simulink model "orbit_propagator_matlab2023b"  (R2023b)
settings: Solver=FixedStepAuto  StartTime=0.0  StopTime=207944  FixedStep=sim_step_size  RelTol=1e-6  AbsTol=1e-7
model workspace (MAT data in the model file):
  current_year = 2025
  year = 2013
values from neighbouring files (symbols this model uses):
  alpha_acc = sqrt(0.7)    [HSat_op_setup_merged_maria.m]    (also in init_orbit_analysis_with_drag_loss.m)
  aph = 200*ones(1,7)    [init_orbit_analysis_with_drag_loss.m]
  COM = [0, 0, 0.25+0.3]    [init_orbit_analysis_with_drag_loss.m]
  ext_ENV_muEarth = 3.986005e14    (= 398600500000000)    [GEO_insertion_setup.m]    (also in HSat_op_setup.m; HSat_op_setup_merged_maria.m; init_orbit_analysis_with_drag_loss.m)
  F107 = 300    [init_orbit_analysis_with_drag_loss.m]
  P_solar = 4.56e-6    (= 4.56e-06)    [HSat_op_setup_merged_maria.m]    (also in init_orbit_analysis_with_drag_loss.m)
  perigee_vector_eci = [0, 1, 0]    [init_orbit_analysis_with_drag_loss.m]
  sim_SC_init_MoI_EOR_wet = [ ... (first row only)    [HSat_op_setup.m]    (also in HSat_op_setup_merged_maria.m; init_orbit_analysis_with_drag_loss.m)
  sim_step_size = 10    [init_orbit_analysis_with_drag_loss.m]
  sun_pointing = 1    [init_orbit_analysis_with_drag_loss.m]
  sun_pointing_SA = 0    [HSat_op_setup_merged_maria.m]    (also in init_orbit_analysis_with_drag_loss.m)
  theta = deg2rad(0)    [init_orbit_analysis_with_drag_loss.m]
undefined symbols (not defined in the file or in its folder): attitude, sun_vector_oc
libraries: aerolibutil x37, matrix_library x37, Toolbox x10, sharedtransform x10, aerolibatmos2 x1, simulink x1, simulink_extras x1
(part 2 of 3)

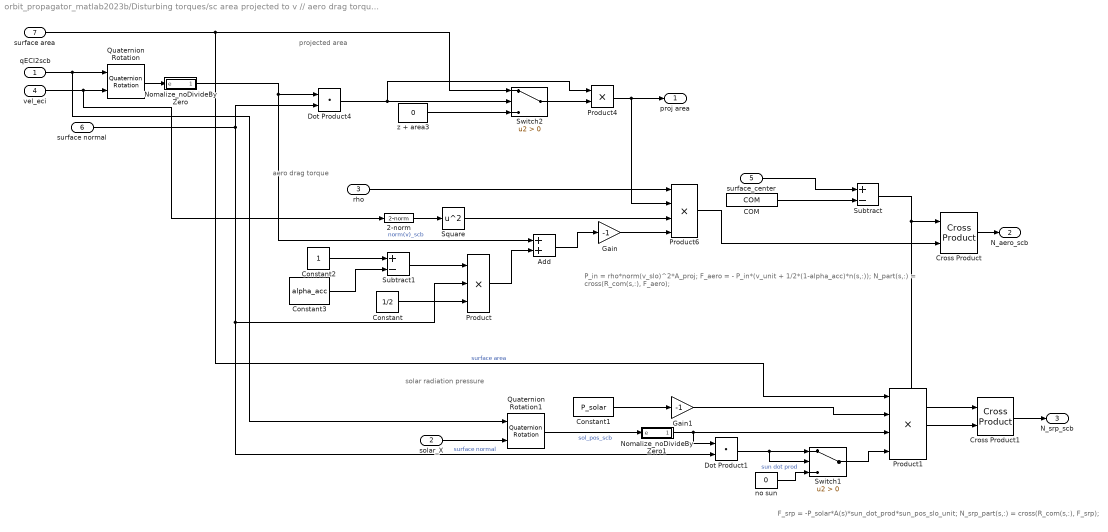
== system orbit_propagator_matlab2023b/Disturbing torques/sc area projected to v // aero drag torque // srp torque/z -6 ==
  note: projected area
  note: aero drag torque
  note: solar radiation pressure
  note: P_in = rho*norm(v_slo)^2*A_proj;
      | F_aero = - P_in*(v_unit + 1/2*(1-alpha_acc)*n(s,:));
      | N_part(s,:) = cross(R_com(s,:), F_aero);
  note: F_srp = -P_solar*A(s)*sun_dot_prod*sun_pos_slo_unit;
      | N_srp_part(s,:) = cross(R_com(s,:), F_srp);
  qECI2scb : Inport
  solar_X : Inport  Port=2
  rho : Inport  Port=3
  vel_eci : Inport  Port=4
  surface_center : Inport  Port=5
  surface normal : Inport  Port=6
  surface area : Inport  Port=7
  2-norm : Toolbox/vector blocks/2-norm  SystemSampleTime=-1  VariantActivationTime=update diagram  AllowFlexibleInterface=on  Latency=0  AutoFrameSizeCalculation=off
      settings: SourceProductName=SSC flight toolbox
  Add : Sum
  COM : Constant  Value=COM
  Constant : Constant  Value=1/2
  Constant1 : Constant  Value=P_solar
  Constant2 : Constant
  Constant3 : Constant  Value=alpha_acc
  Cross Product : matrix_library/Cross Product
  Cross Product1 : matrix_library/Cross Product
  Dot Product1 : DotProduct  OutDataTypeStr=Inherit: Inherit via internal rule
  Dot Product4 : DotProduct  OutDataTypeStr=Inherit: Inherit via internal rule
  Gain : Gain  Gain=-1
  Gain1 : Gain  Gain=-1
  Nomalize_noDivideByZero : Subsystem
      mask Display: disp('u/||u||')
  Nomalize_noDivideByZero1 : Subsystem
      mask Display: disp('u/||u||')
  Product : Product  Inputs=3
  Product1 : Product  Inputs=4
  Product4 : Product
  Product6 : Product  Inputs=4
  Quaternion Rotation : aerolibutil/Quaternion Rotation
  Quaternion Rotation1 : aerolibutil/Quaternion Rotation
  Square : Math  Operator=square
  Subtract : Sum  Inputs=+-
  Subtract1 : Sum  Inputs=+-
  Switch1 : Switch  Criteria=u2 > Threshold  SaturateOnIntegerOverflow=off  InputSameDT=off
  Switch2 : Switch  Criteria=u2 > Threshold  SaturateOnIntegerOverflow=off  InputSameDT=off
  no sun : Constant  Value=0
  z + area3 : Constant  Value=0
  proj area : Outport
  N_aero_scb : Outport  Port=2
  N_srp_scb : Outport  Port=3
  wires:
  Nomalize_noDivideByZero/1(ehat) -> Add/1, Dot Product4/1  "norm(v)_scb"
  surface area/1 -> Product1/1, Switch2/1  "surface area"
  z + area3/1 -> Switch2/3
  Switch2/1 -> Product4/2
  Product4/1 -> Product6/2, proj area/1
  Dot Product4/1 -> Product4/1, Switch2/2
  rho/1 -> Product6/1
  2-norm/1 -> Square/1
  surface normal/1 -> Dot Product4/2, Product/2, Dot Product1/2  "surface normal"
  Constant/1 -> Product/3
  Product/1 -> Add/2
  Gain/1 -> Product6/4
  Product6/1 -> Cross Product/2
  Cross Product/1 -> N_aero_scb/1
  surface_center/1 -> Subtract/1
  COM/1 -> Subtract/2
  Subtract/1 -> Cross Product1/1, Cross Product/1
  Nomalize_noDivideByZero1/1(ehat) -> Product1/3, Dot Product1/1
  Dot Product1/1 -> Switch1/2, Switch1/1  "sun dot prod"
  Constant1/1 -> Gain1/1
  Gain1/1 -> Product1/2
  Product1/1 -> Cross Product1/2
  Cross Product1/1 -> N_srp_scb/1
  vel_eci/1 -> 2-norm/1, Quaternion Rotation/2
  qECI2scb/1 -> Quaternion Rotation1/1, Quaternion Rotation/1
  Quaternion Rotation/1 -> Nomalize_noDivideByZero/1(e)
  solar_X/1 -> Quaternion Rotation1/2
  Quaternion Rotation1/1 -> Nomalize_noDivideByZero1/1(e)  "sol_pos_scb"
  Add/1 -> Gain/1
  Square/1 -> Product6/3
  Switch1/1 -> Product1/4
  no sun/1 -> Switch1/3
  Constant2/1 -> Subtract1/1
  Constant3/1 -> Subtract1/2
  Subtract1/1 -> Product/1

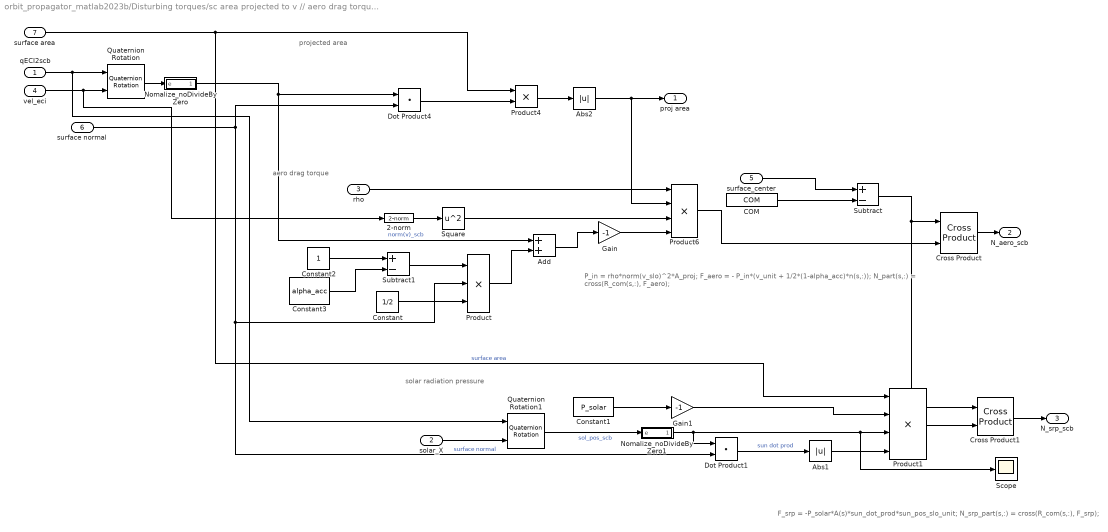
== system orbit_propagator_matlab2023b/Disturbing torques/sc area projected to v // aero drag torque // srp torque/z -7 ==
  note: projected area
  note: aero drag torque
  note: solar radiation pressure
  note: P_in = rho*norm(v_slo)^2*A_proj;
      | F_aero = - P_in*(v_unit + 1/2*(1-alpha_acc)*n(s,:));
      | N_part(s,:) = cross(R_com(s,:), F_aero);
  note: F_srp = -P_solar*A(s)*sun_dot_prod*sun_pos_slo_unit;
      | N_srp_part(s,:) = cross(R_com(s,:), F_srp);
  qECI2scb : Inport
  solar_X : Inport  Port=2
  rho : Inport  Port=3
  vel_eci : Inport  Port=4
  surface_center : Inport  Port=5
  surface normal : Inport  Port=6
  surface area : Inport  Port=7
  2-norm : Toolbox/vector blocks/2-norm  SystemSampleTime=-1  VariantActivationTime=update diagram  AllowFlexibleInterface=on  Latency=0  AutoFrameSizeCalculation=off
      settings: SourceProductName=SSC flight toolbox
  Abs1 : Abs  SaturateOnIntegerOverflow=off
  Abs2 : Abs  SaturateOnIntegerOverflow=off
  Add : Sum
  COM : Constant  Value=COM
  Constant : Constant  Value=1/2
  Constant1 : Constant  Value=P_solar
  Constant2 : Constant
  Constant3 : Constant  Value=alpha_acc
  Cross Product : matrix_library/Cross Product
  Cross Product1 : matrix_library/Cross Product
  Dot Product1 : DotProduct  OutDataTypeStr=Inherit: Inherit via internal rule
  Dot Product4 : DotProduct  OutDataTypeStr=Inherit: Inherit via internal rule
  Gain : Gain  Gain=-1
  Gain1 : Gain  Gain=-1
  Nomalize_noDivideByZero : Subsystem
      mask Display: disp('u/||u||')
  Nomalize_noDivideByZero1 : Subsystem
      mask Display: disp('u/||u||')
  Product : Product  Inputs=3
  Product1 : Product  Inputs=4
  Product4 : Product
  Product6 : Product  Inputs=4
  Quaternion Rotation : aerolibutil/Quaternion Rotation
  Quaternion Rotation1 : aerolibutil/Quaternion Rotation
  Scope : Scope
  Square : Math  Operator=square
  Subtract : Sum  Inputs=+-
  Subtract1 : Sum  Inputs=+-
  proj area : Outport
  N_aero_scb : Outport  Port=2
  N_srp_scb : Outport  Port=3
  wires:
  Nomalize_noDivideByZero/1(ehat) -> Add/1, Dot Product4/1  "norm(v)_scb"
  surface area/1 -> Product4/1, Product1/1  "surface area"
  Product4/1 -> Abs2/1
  Dot Product4/1 -> Product4/2
  rho/1 -> Product6/1
  2-norm/1 -> Square/1
  surface normal/1 -> Dot Product4/2, Product/2, Dot Product1/2  "surface normal"
  Constant/1 -> Product/3
  Product/1 -> Add/2
  Gain/1 -> Product6/4
  Product6/1 -> Cross Product/2
  Cross Product/1 -> N_aero_scb/1
  surface_center/1 -> Subtract/1
  COM/1 -> Subtract/2
  Subtract/1 -> Cross Product1/1, Cross Product/1
  Nomalize_noDivideByZero1/1(ehat) -> Dot Product1/1, Scope/1, Product1/3
  Dot Product1/1 -> Abs1/1  "sun dot prod"
  Constant1/1 -> Gain1/1
  Gain1/1 -> Product1/2
  Product1/1 -> Cross Product1/2
  Cross Product1/1 -> N_srp_scb/1
  vel_eci/1 -> 2-norm/1, Quaternion Rotation/2
  qECI2scb/1 -> Quaternion Rotation1/1, Quaternion Rotation/1
  Quaternion Rotation/1 -> Nomalize_noDivideByZero/1(e)
  solar_X/1 -> Quaternion Rotation1/2
  Quaternion Rotation1/1 -> Nomalize_noDivideByZero1/1(e)  "sol_pos_scb"
  Add/1 -> Gain/1
  Square/1 -> Product6/3
  Constant2/1 -> Subtract1/1
  Constant3/1 -> Subtract1/2
  Subtract1/1 -> Product/1
  Abs2/1 -> Product6/2, proj area/1
  Abs1/1 -> Product1/4

== system orbit_propagator_matlab2023b/Subsystem/Attitude/Att z towards the sun ==
  posECI : Inport
  velECI : Inport  Port=2
  solar_X : Inport  Port=3
  Cross Product : matrix_library/Cross Product
  Cross Product1 : matrix_library/Cross Product
  Cross Product2 : matrix_library/Cross Product
  Direction Cosine Matrix to Quaternions : sharedtransform/Direction Cosine Matrix  to Quaternions  aMode=0  action=None  tolerance=eps(2)
      settings: LibrarySourceBlock=|
      | aerolibtransform2/Direction Cosine Matrix
      | to Quaternions
  Direction Cosine Matrix to Quaternions1 : sharedtransform/Direction Cosine Matrix  to Quaternions  aMode=0  action=Warning  tolerance=eps(2)
      settings: LibrarySourceBlock=|
      | aerolibtransform2/Direction Cosine Matrix
      | to Quaternions
  Matrix Concatenate : Concatenate  NumInputs=3  Mode=Multidimensional array
  Nomalize_noDivideByZero1 : Subsystem
      mask Display: disp('u/||u||')
  Nomalize_noDivideByZero2 : Subsystem
      mask Display: disp('u/||u||')
  Nomalize_noDivideByZero3 : Subsystem
      mask Display: disp('u/||u||')
  Nomalize_noDivideByZero4 : Subsystem
      mask Display: disp('u/||u||')
  Quaternion Multiplication : aerolibutil/Quaternion Multiplication
  rotation matrix around z : Constant  Value=[cos(theta), -sin(theta), 0; sin(theta), cos(theta), 0; 0, 0, 1]
  x : Reshape  OutputDimensionality=Row vector (2-D)
  y : Reshape  OutputDimensionality=Row vector (2-D)
  z : Reshape  OutputDimensionality=Row vector (2-D)
  qECI2scb : Outport
  amECI2scb : Outport  Port=2
  wires:
  posECI/1 -> Cross Product/1  "pos_eci"
  velECI/1 -> Cross Product/2
  z/1 -> Matrix Concatenate/3
  Cross Product1/1 -> Nomalize_noDivideByZero3/1(e)
  Nomalize_noDivideByZero2/1(ehat) -> Cross Product1/1, Cross Product2/1, z/1
  x/1 -> Matrix Concatenate/1
  y/1 -> Matrix Concatenate/2
  Cross Product/1 -> Nomalize_noDivideByZero1/1(e)
  Nomalize_noDivideByZero1/1(ehat) -> Cross Product1/2  "orbit normal"
  Cross Product2/1 -> Nomalize_noDivideByZero4/1(e)
  Matrix Concatenate/1 -> Direction Cosine Matrix to Quaternions/1, amECI2scb/1
  Direction Cosine Matrix to Quaternions/1 -> Quaternion Multiplication/1
  solar_X/1 -> Nomalize_noDivideByZero2/1(e)
  Nomalize_noDivideByZero3/1(ehat) -> Cross Product2/2, x/1
  Nomalize_noDivideByZero4/1(ehat) -> y/1
  rotation matrix around z/1 -> Direction Cosine Matrix to Quaternions1/1
  Direction Cosine Matrix to Quaternions1/1 -> Quaternion Multiplication/2
  Quaternion Multiplication/1 -> qECI2scb/1

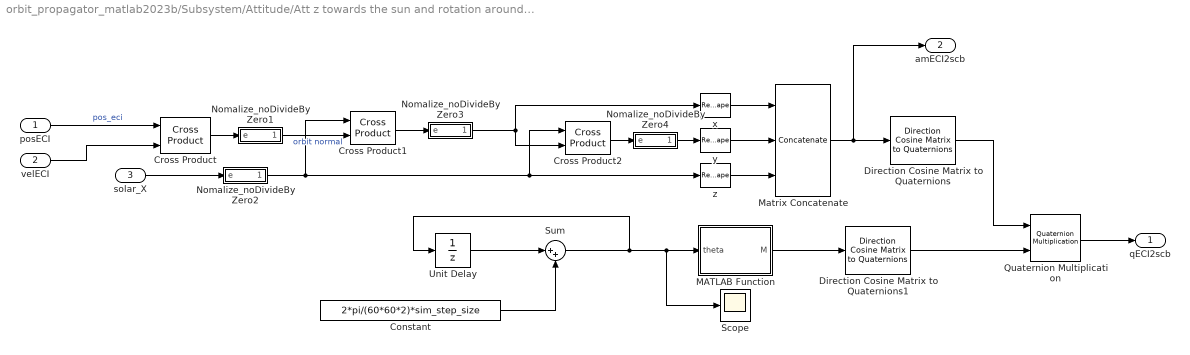
== system orbit_propagator_matlab2023b/Subsystem/Attitude/Att z towards the sun and rotation around z ==
  posECI : Inport
  velECI : Inport  Port=2
  solar_X : Inport  Port=3
  Constant : Constant  Value=2*pi/(60*60*2)*sim_step_size
  Cross Product : matrix_library/Cross Product
  Cross Product1 : matrix_library/Cross Product
  Cross Product2 : matrix_library/Cross Product
  Direction Cosine Matrix to Quaternions : sharedtransform/Direction Cosine Matrix  to Quaternions  aMode=0  action=None  tolerance=eps(2)
      settings: LibrarySourceBlock=|
      | aerolibtransform2/Direction Cosine Matrix
      | to Quaternions
  Direction Cosine Matrix to Quaternions1 : sharedtransform/Direction Cosine Matrix  to Quaternions  aMode=0  action=None  tolerance=eps(2)
      settings: LibrarySourceBlock=|
      | aerolibtransform2/Direction Cosine Matrix
      | to Quaternions
  MATLAB Function : MATLAB Function  TreatAsAtomicUnit=on
  Matrix Concatenate : Concatenate  NumInputs=3  Mode=Multidimensional array
  Nomalize_noDivideByZero1 : Subsystem
      mask Display: disp('u/||u||')
  Nomalize_noDivideByZero2 : Subsystem
      mask Display: disp('u/||u||')
  Nomalize_noDivideByZero3 : Subsystem
      mask Display: disp('u/||u||')
  Nomalize_noDivideByZero4 : Subsystem
      mask Display: disp('u/||u||')
  Quaternion Multiplication : aerolibutil/Quaternion Multiplication
  Scope : Scope
  Sum : Sum  Inputs=|++
  Unit Delay : UnitDelay  SampleTime=-1  HasFrameUpgradeWarning=on
  x : Reshape  OutputDimensionality=Row vector (2-D)
  y : Reshape  OutputDimensionality=Row vector (2-D)
  z : Reshape  OutputDimensionality=Row vector (2-D)
  qECI2scb : Outport
  amECI2scb : Outport  Port=2
  wires:
  posECI/1 -> Cross Product/1  "pos_eci"
  velECI/1 -> Cross Product/2
  z/1 -> Matrix Concatenate/3
  Cross Product1/1 -> Nomalize_noDivideByZero3/1(e)
  Nomalize_noDivideByZero2/1(ehat) -> Cross Product1/1, Cross Product2/1, z/1
  x/1 -> Matrix Concatenate/1
  y/1 -> Matrix Concatenate/2
  Cross Product/1 -> Nomalize_noDivideByZero1/1(e)
  Nomalize_noDivideByZero1/1(ehat) -> Cross Product1/2  "orbit normal"
  Cross Product2/1 -> Nomalize_noDivideByZero4/1(e)
  Matrix Concatenate/1 -> Direction Cosine Matrix to Quaternions/1, amECI2scb/1
  Direction Cosine Matrix to Quaternions/1 -> Quaternion Multiplication/1
  solar_X/1 -> Nomalize_noDivideByZero2/1(e)
  Nomalize_noDivideByZero3/1(ehat) -> Cross Product2/2, x/1
  Nomalize_noDivideByZero4/1(ehat) -> y/1
  MATLAB Function/1(M) -> Direction Cosine Matrix to Quaternions1/1
  Direction Cosine Matrix to Quaternions1/1 -> Quaternion Multiplication/2
  Quaternion Multiplication/1 -> qECI2scb/1
  Unit Delay/1 -> Sum/1
  Constant/1 -> Sum/2
  Sum/1 -> Unit Delay/1, Scope/1, MATLAB Function/1(theta)

== system orbit_propagator_matlab2023b/Subsystem/Attitude/att: z in v ==
  posECI : Inport
  velECI : Inport  Port=2
  Cross Product : matrix_library/Cross Product
  Cross Product1 : matrix_library/Cross Product
  Direction Cosine Matrix to Quaternions : sharedtransform/Direction Cosine Matrix  to Quaternions  aMode=0  action=None  tolerance=eps(2)
      settings: LibrarySourceBlock=|
      | aerolibtransform2/Direction Cosine Matrix
      | to Quaternions
  Matrix Concatenate : Concatenate  NumInputs=3  Mode=Multidimensional array
  Nomalize_noDivideByZero : Subsystem
      mask Display: disp('u/||u||')
  Nomalize_noDivideByZero2 : Subsystem
      mask Display: disp('u/||u||')
  Nomalize_noDivideByZero4 : Subsystem
      mask Display: disp('u/||u||')
  Reshape : Reshape  OutputDimensionality=Row vector (2-D)
  Reshape1 : Reshape  OutputDimensionality=Row vector (2-D)
  Reshape2 : Reshape  OutputDimensionality=Row vector (2-D)
  qECI2scb : Outport  InitialOutput=0
  amECI2scb : Outport  Port=2  InitialOutput=0
  wires:
  posECI/1 -> Nomalize_noDivideByZero/1(e)
  Nomalize_noDivideByZero/1(ehat) -> Cross Product/2
  velECI/1 -> Nomalize_noDivideByZero2/1(e)
  Nomalize_noDivideByZero2/1(ehat) -> Cross Product/1, Cross Product1/2, Reshape2/1  "zslo"
  Cross Product/1 -> Nomalize_noDivideByZero4/1(e)
  Nomalize_noDivideByZero4/1(ehat) -> Cross Product1/1, Reshape1/1  "Yslo"
  Reshape/1 -> Matrix Concatenate/1
  Reshape1/1 -> Matrix Concatenate/2
  Reshape2/1 -> Matrix Concatenate/3
  Direction Cosine Matrix to Quaternions/1 -> qECI2scb/1
  Cross Product1/1 -> Reshape/1
  Matrix Concatenate/1 -> amECI2scb/1, Direction Cosine Matrix to Quaternions/1

== system orbit_propagator_matlab2023b/Subsystem/Attitude/changes with altitude ==
  posECI : Inport
  velECI : Inport  Port=2
  1 z in v 0 x in v : Constant  Value=attitude
  2-norm : Toolbox/vector blocks/2-norm  SystemSampleTime=-1  VariantActivationTime=update diagram  Latency=0  AutoFrameSizeCalculation=off
      settings: SourceProductName=SSC flight toolbox
  Constant : Constant
  Constant1 : Constant  Value=0
  If : If  IfExpression=u1 < 7.2e6
  If Action Subsystem : Subsystem  TreatAsAtomicUnit=on
  If Action Subsystem1 : Subsystem  TreatAsAtomicUnit=on
      settings: LibrarySourceBlock=|
      | hdlsllib/Ports &
      | Subsystems/If Action
      | Subsystem
  Merge : Merge
  Switch{,1..3} (4 alike) : Switch  Criteria=u2 > Threshold  SaturateOnIntegerOverflow=off  InputSameDT=off
  q (x in v) : Subsystem
  q (z in r) : Subsystem
  q (z in v) : Subsystem
  qECI2scb : Outport
  amECI2scb : Outport  Port=2
  wires:
  q (z in r)/1(qECI2slor) -> Switch1/3
  posECI/1 -> 2-norm/1, q (z in r)/1(posECI), q (x in v)/1(posECI), q (z in v)/1(posECI)  "pos_eci"
  q (z in r)/2(amECI2slor1) -> Switch/3
  Constant/1 -> If Action Subsystem/1(In1)
  Constant1/1 -> If Action Subsystem1/1(In1)
  If Action Subsystem/1(Out1) -> Merge/1
  If Action Subsystem1/1(Out1) -> Merge/2
  Merge/1 -> Switch1/2, Switch/2
  Switch1/1 -> qECI2scb/1
  Switch/1 -> amECI2scb/1
  1 z in v 0 x in v/1 -> Switch3/2, Switch2/2
  q (z in v)/1(qECI2scbv) -> Switch2/1
  q (z in v)/2(amECI2scbv) -> Switch3/1
  q (x in v)/1(qECI2scb) -> Switch2/3
  q (x in v)/2(amECI2slov1) -> Switch3/3
  Switch2/1 -> Switch1/1
  Switch3/1 -> Switch/1
  2-norm/1 -> If/1
  If/1 -> If Action Subsystem/Action
  If/2 -> If Action Subsystem1/Action
  velECI/1 -> q (z in v)/2(velECI), q (x in v)/2(velECI), q (z in r)/2(velECI)

== system orbit_propagator_matlab2023b/Subsystem/Attitude/q (z in r) ==
  note: sc_z=-T_pos(ii,:)/norm(T_pos(ii,:));
      | sc_y=cross(sc_z,T_vel(ii,:));
      | sc_y=sc_y/norm(sc_y);
      | sc_x=cross(sc_y,sc_z);
      | sc_x=sc_x/norm(sc_x);
  posECI : Inport
  velECI : Inport  Port=2
  -1 : Gain  Gain=-1
  Cross Product : matrix_library/Cross Product
  Cross Product1 : matrix_library/Cross Product
  Direction Cosine Matrix to Quaternions : sharedtransform/Direction Cosine Matrix  to Quaternions  aMode=0  action=None  tolerance=eps(2)
      settings: LibrarySourceBlock=|
      | aerolibtransform2/Direction Cosine Matrix
      | to Quaternions
  Matrix Concatenate : Concatenate  NumInputs=3  Mode=Multidimensional array
  Nomalize_noDivideByZero : Subsystem
      mask Display: disp('u/||u||')
  Nomalize_noDivideByZero2 : Subsystem
      mask Display: disp('u/||u||')
  Nomalize_noDivideByZero4 : Subsystem
      mask Display: disp('u/||u||')
  x : Reshape  OutputDimensionality=Row vector (2-D)
  y : Reshape  OutputDimensionality=Row vector (2-D)
  z : Reshape  OutputDimensionality=Row vector (2-D)
  qECI2scb : Outport  InitialOutput=0
  amECI2scb : Outport  Port=2  InitialOutput=0
  wires:
  -1/1 -> Cross Product1/2, z/1, Cross Product/1  "Zslo"
  posECI/1 -> Nomalize_noDivideByZero/1(e)
  Nomalize_noDivideByZero/1(ehat) -> -1/1
  velECI/1 -> Nomalize_noDivideByZero2/1(e)
  Nomalize_noDivideByZero2/1(ehat) -> Cross Product/2
  Cross Product/1 -> Nomalize_noDivideByZero4/1(e)
  Nomalize_noDivideByZero4/1(ehat) -> Cross Product1/1, y/1  "Yslo"
  Cross Product1/1 -> x/1
  x/1 -> Matrix Concatenate/1
  y/1 -> Matrix Concatenate/2
  z/1 -> Matrix Concatenate/3
  Direction Cosine Matrix to Quaternions/1 -> qECI2scb/1
  Matrix Concatenate/1 -> amECI2scb/1, Direction Cosine Matrix to Quaternions/1

== system orbit_propagator_matlab2023b/Subsystem/sun pointing in orbit plane/Nomalize_noDivideByZero1 ==
  e : Inport
  2-norm : Subsystem
      mask Display: disp('||u||')
  Product : Product  Inputs=*/  InputSameDT=on  RndMeth=Zero  SaturateOnIntegerOverflow=on  OutDataTypeStr=Inherit: Same as first input
  Switch : Switch  Criteria=u2 > Threshold  SaturateOnIntegerOverflow=off  InputSameDT=off
  zero : Constant  Value=0
  ehat : Outport
  wires:
  e/1 -> 2-norm/1(In1), Product/1
  2-norm/1(Out1) -> Switch/2, Product/2
  Switch/1 -> ehat/1
  Product/1 -> Switch/1
  zero/1 -> Switch/3

== system orbit_propagator_matlab2023b/Subsystem/sun pointing in orbit plane/Nomalize_noDivideByZero3 ==
  e : Inport
  2-norm : Subsystem
      mask Display: disp('||u||')
  Product : Product  Inputs=*/  InputSameDT=on  RndMeth=Zero  SaturateOnIntegerOverflow=on  OutDataTypeStr=Inherit: Same as first input
  Switch : Switch  Criteria=u2 > Threshold  SaturateOnIntegerOverflow=off  InputSameDT=off
  zero : Constant  Value=0
  ehat : Outport
  wires:
  e/1 -> 2-norm/1(In1), Product/1
  2-norm/1(Out1) -> Switch/2, Product/2
  Switch/1 -> ehat/1
  Product/1 -> Switch/1
  zero/1 -> Switch/3

== system orbit_propagator_matlab2023b/spare systems/Subsystem/within sight ==
  pos_ecef : Inport
  "GS long, lat (deg)" : Inport  Port=2
  view angle : Inport  Port=3
  2-norm : Toolbox/vector blocks/2-norm  SystemSampleTime=-1  VariantActivationTime=update diagram  Latency=0  AutoFrameSizeCalculation=off
      settings: SourceProductName=SSC flight toolbox
  2-norm1 : Toolbox/vector blocks/2-norm  SystemSampleTime=-1  VariantActivationTime=update diagram  Latency=0  AutoFrameSizeCalculation=off
      settings: SourceProductName=SSC flight toolbox
  Acos : Trigonometry  Operator=acos
  Compare To Zero : simulink/Logic and Bit Operations/Compare To Zero  relop=>  OutDataTypeStr=boolean
  Constant : Constant  Value=0
  Degrees to Radians : simulink_extras/Transformations/Degrees to Radians
  Divide : Product  Inputs=*//
  Dot Product : DotProduct  OutDataTypeStr=Inherit: Inherit via internal rule
  LLA to ECEF Position : LLA2ECEF
  Subtract : Sum  Inputs=+-
  within sight boolean : Outport
  wires:
  "GS long, lat (deg)"/1 -> LLA to ECEF Position/1
  Constant/1 -> LLA to ECEF Position/2
  LLA to ECEF Position/1 -> 2-norm/1, Dot Product/2
  pos_ecef/1 -> 2-norm1/1, Dot Product/1
  Dot Product/1 -> Divide/1
  2-norm/1 -> Divide/2
  2-norm1/1 -> Divide/3
  Divide/1 -> Acos/1
  view angle/1 -> Degrees to Radians/1
  Degrees to Radians/1 -> Subtract/1
  Acos/1 -> Subtract/2
  Subtract/1 -> Compare To Zero/1
  Compare To Zero/1 -> within sight boolean/1

== system orbit_propagator_matlab2023b/spare systems/create custom sun vector/Nomalize_noDivideByZero1 ==
  e : Inport
  2-norm : Subsystem
      mask Display: disp('||u||')
  Product : Product  Inputs=*/  InputSameDT=on  RndMeth=Zero  SaturateOnIntegerOverflow=on  OutDataTypeStr=Inherit: Same as first input
  Switch : Switch  Criteria=u2 > Threshold  SaturateOnIntegerOverflow=off  InputSameDT=off
  zero : Constant  Value=0
  ehat : Outport
  wires:
  e/1 -> 2-norm/1(In1), Product/1
  2-norm/1(Out1) -> Switch/2, Product/2
  Switch/1 -> ehat/1
  Product/1 -> Switch/1
  zero/1 -> Switch/3

== system orbit_propagator_matlab2023b/spare systems/create custom sun vector/Nomalize_noDivideByZero2 ==
  e : Inport
  2-norm : Subsystem
      mask Display: disp('||u||')
  Product : Product  Inputs=*/  InputSameDT=on  RndMeth=Zero  SaturateOnIntegerOverflow=on  OutDataTypeStr=Inherit: Same as first input
  Switch : Switch  Criteria=u2 > Threshold  SaturateOnIntegerOverflow=off  InputSameDT=off
  zero : Constant  Value=0
  ehat : Outport
  wires:
  e/1 -> 2-norm/1(In1), Product/1
  2-norm/1(Out1) -> Switch/2, Product/2
  Switch/1 -> ehat/1
  Product/1 -> Switch/1
  zero/1 -> Switch/3

== system orbit_propagator_matlab2023b/spare systems/sun_angle_slo/Nomalize_noDivideByZero ==
  e : Inport
  2-norm : Subsystem
      mask Display: disp('||u||')
  Product : Product  Inputs=*/  InputSameDT=on  RndMeth=Zero  SaturateOnIntegerOverflow=on  OutDataTypeStr=Inherit: Same as first input
  Switch : Switch  Criteria=u2 > Threshold  SaturateOnIntegerOverflow=off  InputSameDT=off
  zero : Constant  Value=0
  ehat : Outport
  wires:
  e/1 -> 2-norm/1(In1), Product/1
  2-norm/1(Out1) -> Switch/2, Product/2
  Switch/1 -> ehat/1
  Product/1 -> Switch/1
  zero/1 -> Switch/3

== system orbit_propagator_matlab2023b/Disturbing torques/sc area projected to v // aero drag torque // srp torque/Switch Case Action Subsystem/sun pointing solar arrays ==
  SC2sun_eci : Inport
  qECI2scb : Inport  Port=2
  Constant2 : Constant  Value=[1, 0, 1]
  Nomalize_noDivideByZero1 : Subsystem
      mask Display: disp('u/||u||')
  Product2 : Product
  Quaternion Rotation2 : aerolibutil/Quaternion Rotation
  SA normal : Outport
  wires:
  qECI2scb/1 -> Quaternion Rotation2/1
  SC2sun_eci/1 -> Quaternion Rotation2/2
  Quaternion Rotation2/1 -> Product2/1  "sun pos scb"
  Constant2/1 -> Product2/2
  Product2/1 -> Nomalize_noDivideByZero1/1(e)
  Nomalize_noDivideByZero1/1(ehat) -> SA normal/1  "surface normal scb"

== system orbit_propagator_matlab2023b/Disturbing torques/sc area projected to v // aero drag torque // srp torque/z -1/Nomalize_noDivideByZero ==
  e : Inport
  2-norm : Subsystem
      mask Display: disp('||u||')
  Product : Product  Inputs=*/  InputSameDT=on  RndMeth=Zero  SaturateOnIntegerOverflow=on  OutDataTypeStr=Inherit: Same as first input
  Switch : Switch  Criteria=u2 > Threshold  SaturateOnIntegerOverflow=off  InputSameDT=off
  zero : Constant  Value=0
  ehat : Outport
  wires:
  e/1 -> 2-norm/1(In1), Product/1
  2-norm/1(Out1) -> Switch/2, Product/2
  Switch/1 -> ehat/1
  Product/1 -> Switch/1
  zero/1 -> Switch/3

== system orbit_propagator_matlab2023b/Disturbing torques/sc area projected to v // aero drag torque // srp torque/z -1/Nomalize_noDivideByZero1 ==
  e : Inport
  2-norm : Subsystem
      mask Display: disp('||u||')
  Product : Product  Inputs=*/  InputSameDT=on  RndMeth=Zero  SaturateOnIntegerOverflow=on  OutDataTypeStr=Inherit: Same as first input
  Switch : Switch  Criteria=u2 > Threshold  SaturateOnIntegerOverflow=off  InputSameDT=off
  zero : Constant  Value=0
  ehat : Outport
  wires:
  e/1 -> 2-norm/1(In1), Product/1
  2-norm/1(Out1) -> Switch/2, Product/2
  Switch/1 -> ehat/1
  Product/1 -> Switch/1
  zero/1 -> Switch/3

== system orbit_propagator_matlab2023b/Disturbing torques/sc area projected to v // aero drag torque // srp torque/z -2/Nomalize_noDivideByZero ==
  e : Inport
  2-norm : Subsystem
      mask Display: disp('||u||')
  Product : Product  Inputs=*/  InputSameDT=on  RndMeth=Zero  SaturateOnIntegerOverflow=on  OutDataTypeStr=Inherit: Same as first input
  Switch : Switch  Criteria=u2 > Threshold  SaturateOnIntegerOverflow=off  InputSameDT=off
  zero : Constant  Value=0
  ehat : Outport
  wires:
  e/1 -> 2-norm/1(In1), Product/1
  2-norm/1(Out1) -> Switch/2, Product/2
  Switch/1 -> ehat/1
  Product/1 -> Switch/1
  zero/1 -> Switch/3

== system orbit_propagator_matlab2023b/Disturbing torques/sc area projected to v // aero drag torque // srp torque/z -2/Nomalize_noDivideByZero1 ==
  e : Inport
  2-norm : Subsystem
      mask Display: disp('||u||')
  Product : Product  Inputs=*/  InputSameDT=on  RndMeth=Zero  SaturateOnIntegerOverflow=on  OutDataTypeStr=Inherit: Same as first input
  Switch : Switch  Criteria=u2 > Threshold  SaturateOnIntegerOverflow=off  InputSameDT=off
  zero : Constant  Value=0
  ehat : Outport
  wires:
  e/1 -> 2-norm/1(In1), Product/1
  2-norm/1(Out1) -> Switch/2, Product/2
  Switch/1 -> ehat/1
  Product/1 -> Switch/1
  zero/1 -> Switch/3

== system orbit_propagator_matlab2023b/Disturbing torques/sc area projected to v // aero drag torque // srp torque/z -3/Nomalize_noDivideByZero ==
  e : Inport
  2-norm : Subsystem
      mask Display: disp('||u||')
  Product : Product  Inputs=*/  InputSameDT=on  RndMeth=Zero  SaturateOnIntegerOverflow=on  OutDataTypeStr=Inherit: Same as first input
  Switch : Switch  Criteria=u2 > Threshold  SaturateOnIntegerOverflow=off  InputSameDT=off
  zero : Constant  Value=0
  ehat : Outport
  wires:
  e/1 -> 2-norm/1(In1), Product/1
  2-norm/1(Out1) -> Switch/2, Product/2
  Switch/1 -> ehat/1
  Product/1 -> Switch/1
  zero/1 -> Switch/3

== system orbit_propagator_matlab2023b/Disturbing torques/sc area projected to v // aero drag torque // srp torque/z -3/Nomalize_noDivideByZero1 ==
  e : Inport
  2-norm : Subsystem
      mask Display: disp('||u||')
  Product : Product  Inputs=*/  InputSameDT=on  RndMeth=Zero  SaturateOnIntegerOverflow=on  OutDataTypeStr=Inherit: Same as first input
  Switch : Switch  Criteria=u2 > Threshold  SaturateOnIntegerOverflow=off  InputSameDT=off
  zero : Constant  Value=0
  ehat : Outport
  wires:
  e/1 -> 2-norm/1(In1), Product/1
  2-norm/1(Out1) -> Switch/2, Product/2
  Switch/1 -> ehat/1
  Product/1 -> Switch/1
  zero/1 -> Switch/3

== system orbit_propagator_matlab2023b/Disturbing torques/sc area projected to v // aero drag torque // srp torque/z -4/Nomalize_noDivideByZero ==
  e : Inport
  2-norm : Subsystem
      mask Display: disp('||u||')
  Product : Product  Inputs=*/  InputSameDT=on  RndMeth=Zero  SaturateOnIntegerOverflow=on  OutDataTypeStr=Inherit: Same as first input
  Switch : Switch  Criteria=u2 > Threshold  SaturateOnIntegerOverflow=off  InputSameDT=off
  zero : Constant  Value=0
  ehat : Outport
  wires:
  e/1 -> 2-norm/1(In1), Product/1
  2-norm/1(Out1) -> Switch/2, Product/2
  Switch/1 -> ehat/1
  Product/1 -> Switch/1
  zero/1 -> Switch/3

== system orbit_propagator_matlab2023b/Disturbing torques/sc area projected to v // aero drag torque // srp torque/z -4/Nomalize_noDivideByZero1 ==
  e : Inport
  2-norm : Subsystem
      mask Display: disp('||u||')
  Product : Product  Inputs=*/  InputSameDT=on  RndMeth=Zero  SaturateOnIntegerOverflow=on  OutDataTypeStr=Inherit: Same as first input
  Switch : Switch  Criteria=u2 > Threshold  SaturateOnIntegerOverflow=off  InputSameDT=off
  zero : Constant  Value=0
  ehat : Outport
  wires:
  e/1 -> 2-norm/1(In1), Product/1
  2-norm/1(Out1) -> Switch/2, Product/2
  Switch/1 -> ehat/1
  Product/1 -> Switch/1
  zero/1 -> Switch/3

== system orbit_propagator_matlab2023b/Disturbing torques/sc area projected to v // aero drag torque // srp torque/z -5/Nomalize_noDivideByZero ==
  e : Inport
  2-norm : Subsystem
      mask Display: disp('||u||')
  Product : Product  Inputs=*/  InputSameDT=on  RndMeth=Zero  SaturateOnIntegerOverflow=on  OutDataTypeStr=Inherit: Same as first input
  Switch : Switch  Criteria=u2 > Threshold  SaturateOnIntegerOverflow=off  InputSameDT=off
  zero : Constant  Value=0
  ehat : Outport
  wires:
  e/1 -> 2-norm/1(In1), Product/1
  2-norm/1(Out1) -> Switch/2, Product/2
  Switch/1 -> ehat/1
  Product/1 -> Switch/1
  zero/1 -> Switch/3

== system orbit_propagator_matlab2023b/Disturbing torques/sc area projected to v // aero drag torque // srp torque/z -5/Nomalize_noDivideByZero1 ==
  e : Inport
  2-norm : Subsystem
      mask Display: disp('||u||')
  Product : Product  Inputs=*/  InputSameDT=on  RndMeth=Zero  SaturateOnIntegerOverflow=on  OutDataTypeStr=Inherit: Same as first input
  Switch : Switch  Criteria=u2 > Threshold  SaturateOnIntegerOverflow=off  InputSameDT=off
  zero : Constant  Value=0
  ehat : Outport
  wires:
  e/1 -> 2-norm/1(In1), Product/1
  2-norm/1(Out1) -> Switch/2, Product/2
  Switch/1 -> ehat/1
  Product/1 -> Switch/1
  zero/1 -> Switch/3

== system orbit_propagator_matlab2023b/Disturbing torques/sc area projected to v // aero drag torque // srp torque/z -6/Nomalize_noDivideByZero ==
  e : Inport
  2-norm : Subsystem
      mask Display: disp('||u||')
  Product : Product  Inputs=*/  InputSameDT=on  RndMeth=Zero  SaturateOnIntegerOverflow=on  OutDataTypeStr=Inherit: Same as first input
  Switch : Switch  Criteria=u2 > Threshold  SaturateOnIntegerOverflow=off  InputSameDT=off
  zero : Constant  Value=0
  ehat : Outport
  wires:
  e/1 -> 2-norm/1(In1), Product/1
  2-norm/1(Out1) -> Switch/2, Product/2
  Switch/1 -> ehat/1
  Product/1 -> Switch/1
  zero/1 -> Switch/3

== system orbit_propagator_matlab2023b/Disturbing torques/sc area projected to v // aero drag torque // srp torque/z -6/Nomalize_noDivideByZero1 ==
  e : Inport
  2-norm : Subsystem
      mask Display: disp('||u||')
  Product : Product  Inputs=*/  InputSameDT=on  RndMeth=Zero  SaturateOnIntegerOverflow=on  OutDataTypeStr=Inherit: Same as first input
  Switch : Switch  Criteria=u2 > Threshold  SaturateOnIntegerOverflow=off  InputSameDT=off
  zero : Constant  Value=0
  ehat : Outport
  wires:
  e/1 -> 2-norm/1(In1), Product/1
  2-norm/1(Out1) -> Switch/2, Product/2
  Switch/1 -> ehat/1
  Product/1 -> Switch/1
  zero/1 -> Switch/3

== system orbit_propagator_matlab2023b/Disturbing torques/sc area projected to v // aero drag torque // srp torque/z -7/Nomalize_noDivideByZero ==
  e : Inport
  2-norm : Subsystem
      mask Display: disp('||u||')
  Product : Product  Inputs=*/  InputSameDT=on  RndMeth=Zero  SaturateOnIntegerOverflow=on  OutDataTypeStr=Inherit: Same as first input
  Switch : Switch  Criteria=u2 > Threshold  SaturateOnIntegerOverflow=off  InputSameDT=off
  zero : Constant  Value=0
  ehat : Outport
  wires:
  e/1 -> 2-norm/1(In1), Product/1
  2-norm/1(Out1) -> Switch/2, Product/2
  Switch/1 -> ehat/1
  Product/1 -> Switch/1
  zero/1 -> Switch/3

== system orbit_propagator_matlab2023b/Disturbing torques/sc area projected to v // aero drag torque // srp torque/z -7/Nomalize_noDivideByZero1 ==
  e : Inport
  2-norm : Subsystem
      mask Display: disp('||u||')
  Product : Product  Inputs=*/  InputSameDT=on  RndMeth=Zero  SaturateOnIntegerOverflow=on  OutDataTypeStr=Inherit: Same as first input
  Switch : Switch  Criteria=u2 > Threshold  SaturateOnIntegerOverflow=off  InputSameDT=off
  zero : Constant  Value=0
  ehat : Outport
  wires:
  e/1 -> 2-norm/1(In1), Product/1
  2-norm/1(Out1) -> Switch/2, Product/2
  Switch/1 -> ehat/1
  Product/1 -> Switch/1
  zero/1 -> Switch/3

== system orbit_propagator_matlab2023b/Subsystem/Attitude/Att z towards the sun/Nomalize_noDivideByZero1 ==
  e : Inport
  2-norm : Subsystem
      mask Display: disp('||u||')
  Product : Product  Inputs=*/  InputSameDT=on  RndMeth=Zero  SaturateOnIntegerOverflow=on  OutDataTypeStr=Inherit: Same as first input
  Switch : Switch  Criteria=u2 > Threshold  SaturateOnIntegerOverflow=off  InputSameDT=off
  zero : Constant  Value=0
  ehat : Outport
  wires:
  e/1 -> 2-norm/1(In1), Product/1
  2-norm/1(Out1) -> Switch/2, Product/2
  Switch/1 -> ehat/1
  Product/1 -> Switch/1
  zero/1 -> Switch/3

== system orbit_propagator_matlab2023b/Subsystem/Attitude/Att z towards the sun/Nomalize_noDivideByZero2 ==
  e : Inport
  2-norm : Subsystem
      mask Display: disp('||u||')
  Product : Product  Inputs=*/  InputSameDT=on  RndMeth=Zero  SaturateOnIntegerOverflow=on  OutDataTypeStr=Inherit: Same as first input
  Switch : Switch  Criteria=u2 > Threshold  SaturateOnIntegerOverflow=off  InputSameDT=off
  zero : Constant  Value=0
  ehat : Outport
  wires:
  e/1 -> 2-norm/1(In1), Product/1
  2-norm/1(Out1) -> Switch/2, Product/2
  Switch/1 -> ehat/1
  Product/1 -> Switch/1
  zero/1 -> Switch/3

== system orbit_propagator_matlab2023b/Subsystem/Attitude/Att z towards the sun/Nomalize_noDivideByZero3 ==
  e : Inport
  2-norm : Subsystem
      mask Display: disp('||u||')
  Product : Product  Inputs=*/  InputSameDT=on  RndMeth=Zero  SaturateOnIntegerOverflow=on  OutDataTypeStr=Inherit: Same as first input
  Switch : Switch  Criteria=u2 > Threshold  SaturateOnIntegerOverflow=off  InputSameDT=off
  zero : Constant  Value=0
  ehat : Outport
  wires:
  e/1 -> 2-norm/1(In1), Product/1
  2-norm/1(Out1) -> Switch/2, Product/2
  Switch/1 -> ehat/1
  Product/1 -> Switch/1
  zero/1 -> Switch/3

== system orbit_propagator_matlab2023b/Subsystem/Attitude/Att z towards the sun/Nomalize_noDivideByZero4 ==
  e : Inport
  2-norm : Subsystem
      mask Display: disp('||u||')
  Product : Product  Inputs=*/  InputSameDT=on  RndMeth=Zero  SaturateOnIntegerOverflow=on  OutDataTypeStr=Inherit: Same as first input
  Switch : Switch  Criteria=u2 > Threshold  SaturateOnIntegerOverflow=off  InputSameDT=off
  zero : Constant  Value=0
  ehat : Outport
  wires:
  e/1 -> 2-norm/1(In1), Product/1
  2-norm/1(Out1) -> Switch/2, Product/2
  Switch/1 -> ehat/1
  Product/1 -> Switch/1
  zero/1 -> Switch/3

== system orbit_propagator_matlab2023b/Subsystem/Attitude/Att z towards the sun and rotation around z/Nomalize_noDivideByZero1 ==
  e : Inport
  2-norm : Subsystem
      mask Display: disp('||u||')
  Product : Product  Inputs=*/  InputSameDT=on  RndMeth=Zero  SaturateOnIntegerOverflow=on  OutDataTypeStr=Inherit: Same as first input
  Switch : Switch  Criteria=u2 > Threshold  SaturateOnIntegerOverflow=off  InputSameDT=off
  zero : Constant  Value=0
  ehat : Outport
  wires:
  e/1 -> 2-norm/1(In1), Product/1
  2-norm/1(Out1) -> Switch/2, Product/2
  Switch/1 -> ehat/1
  Product/1 -> Switch/1
  zero/1 -> Switch/3

== system orbit_propagator_matlab2023b/Subsystem/Attitude/Att z towards the sun and rotation around z/Nomalize_noDivideByZero2 ==
  e : Inport
  2-norm : Subsystem
      mask Display: disp('||u||')
  Product : Product  Inputs=*/  InputSameDT=on  RndMeth=Zero  SaturateOnIntegerOverflow=on  OutDataTypeStr=Inherit: Same as first input
  Switch : Switch  Criteria=u2 > Threshold  SaturateOnIntegerOverflow=off  InputSameDT=off
  zero : Constant  Value=0
  ehat : Outport
  wires:
  e/1 -> 2-norm/1(In1), Product/1
  2-norm/1(Out1) -> Switch/2, Product/2
  Switch/1 -> ehat/1
  Product/1 -> Switch/1
  zero/1 -> Switch/3

== system orbit_propagator_matlab2023b/Subsystem/Attitude/Att z towards the sun and rotation around z/Nomalize_noDivideByZero3 ==
  e : Inport
  2-norm : Subsystem
      mask Display: disp('||u||')
  Product : Product  Inputs=*/  InputSameDT=on  RndMeth=Zero  SaturateOnIntegerOverflow=on  OutDataTypeStr=Inherit: Same as first input
  Switch : Switch  Criteria=u2 > Threshold  SaturateOnIntegerOverflow=off  InputSameDT=off
  zero : Constant  Value=0
  ehat : Outport
  wires:
  e/1 -> 2-norm/1(In1), Product/1
  2-norm/1(Out1) -> Switch/2, Product/2
  Switch/1 -> ehat/1
  Product/1 -> Switch/1
  zero/1 -> Switch/3

== system orbit_propagator_matlab2023b/Subsystem/Attitude/Att z towards the sun and rotation around z/Nomalize_noDivideByZero4 ==
  e : Inport
  2-norm : Subsystem
      mask Display: disp('||u||')
  Product : Product  Inputs=*/  InputSameDT=on  RndMeth=Zero  SaturateOnIntegerOverflow=on  OutDataTypeStr=Inherit: Same as first input
  Switch : Switch  Criteria=u2 > Threshold  SaturateOnIntegerOverflow=off  InputSameDT=off
  zero : Constant  Value=0
  ehat : Outport
  wires:
  e/1 -> 2-norm/1(In1), Product/1
  2-norm/1(Out1) -> Switch/2, Product/2
  Switch/1 -> ehat/1
  Product/1 -> Switch/1
  zero/1 -> Switch/3

== system orbit_propagator_matlab2023b/Subsystem/Attitude/att: z in v/Nomalize_noDivideByZero ==
  e : Inport
  2-norm : Subsystem
      mask Display: disp('||u||')
  Product : Product  Inputs=*/  InputSameDT=on  RndMeth=Zero  SaturateOnIntegerOverflow=on  OutDataTypeStr=Inherit: Same as first input
  Switch : Switch  Criteria=u2 > Threshold  SaturateOnIntegerOverflow=off  InputSameDT=off
  zero : Constant  Value=0
  ehat : Outport
  wires:
  e/1 -> 2-norm/1(In1), Product/1
  2-norm/1(Out1) -> Switch/2, Product/2
  Switch/1 -> ehat/1
  Product/1 -> Switch/1
  zero/1 -> Switch/3

== system orbit_propagator_matlab2023b/Subsystem/Attitude/att: z in v/Nomalize_noDivideByZero2 ==
  e : Inport
  2-norm : Subsystem
      mask Display: disp('||u||')
  Product : Product  Inputs=*/  InputSameDT=on  RndMeth=Zero  SaturateOnIntegerOverflow=on  OutDataTypeStr=Inherit: Same as first input
  Switch : Switch  Criteria=u2 > Threshold  SaturateOnIntegerOverflow=off  InputSameDT=off
  zero : Constant  Value=0
  ehat : Outport
  wires:
  e/1 -> 2-norm/1(In1), Product/1
  2-norm/1(Out1) -> Switch/2, Product/2
  Switch/1 -> ehat/1
  Product/1 -> Switch/1
  zero/1 -> Switch/3

== system orbit_propagator_matlab2023b/Subsystem/Attitude/att: z in v/Nomalize_noDivideByZero4 ==
  e : Inport
  2-norm : Subsystem
      mask Display: disp('||u||')
  Product : Product  Inputs=*/  InputSameDT=on  RndMeth=Zero  SaturateOnIntegerOverflow=on  OutDataTypeStr=Inherit: Same as first input
  Switch : Switch  Criteria=u2 > Threshold  SaturateOnIntegerOverflow=off  InputSameDT=off
  zero : Constant  Value=0
  ehat : Outport
  wires:
  e/1 -> 2-norm/1(In1), Product/1
  2-norm/1(Out1) -> Switch/2, Product/2
  Switch/1 -> ehat/1
  Product/1 -> Switch/1
  zero/1 -> Switch/3

== system orbit_propagator_matlab2023b/Subsystem/Attitude/changes with altitude/If Action Subsystem ==
  In1 : Inport
  Action Port : ActionPort
  Out1 : Outport
  wires:
  In1/1 -> Out1/1

== system orbit_propagator_matlab2023b/Subsystem/Attitude/changes with altitude/If Action Subsystem1 ==
  In1 : Inport
  Action Port : ActionPort
  Out1 : Outport
  wires:
  In1/1 -> Out1/1

== system orbit_propagator_matlab2023b/Subsystem/Attitude/changes with altitude/q (x in v) ==
  posECI : Inport
  velECI : Inport  Port=2
  Cross Product1 : matrix_library/Cross Product
  Cross Product2 : matrix_library/Cross Product
  Direction Cosine Matrix to Quaternions : sharedtransform/Direction Cosine Matrix  to Quaternions  aMode=0  action=Warning  tolerance=eps(2)
      settings: LibrarySourceBlock=|
      | aerolibtransform2/Direction Cosine Matrix
      | to Quaternions
  Matrix Concatenate : Concatenate  NumInputs=3  Mode=Multidimensional array
  Nomalize_noDivideByZero : Subsystem
      mask Display: disp('u/||u||')
  Nomalize_noDivideByZero1 : Subsystem
      mask Display: disp('u/||u||')
  Nomalize_noDivideByZero2 : Subsystem
      mask Display: disp('u/||u||')
  Nomalize_noDivideByZero4 : Subsystem
      mask Display: disp('u/||u||')
  Reshape : Reshape  OutputDimensionality=Row vector (2-D)
  Reshape1 : Reshape  OutputDimensionality=Row vector (2-D)
  Reshape2 : Reshape  OutputDimensionality=Row vector (2-D)
  qECI2scb : Outport  InitialOutput=0
  amECI2slov1 : Outport  Port=2  InitialOutput=0
  wires:
  posECI/1 -> Nomalize_noDivideByZero/1(e)
  velECI/1 -> Nomalize_noDivideByZero2/1(e)
  Cross Product1/1 -> Nomalize_noDivideByZero4/1(e)
  Nomalize_noDivideByZero4/1(ehat) -> Cross Product2/2, Reshape1/1  "Y"
  Reshape/1 -> Matrix Concatenate/1
  Reshape1/1 -> Matrix Concatenate/2
  Direction Cosine Matrix to Quaternions/1 -> qECI2scb/1
  Cross Product2/1 -> Nomalize_noDivideByZero1/1(e)
  Matrix Concatenate/1 -> Direction Cosine Matrix to Quaternions/1, amECI2slov1/1
  Nomalize_noDivideByZero2/1(ehat) -> Cross Product2/1, Cross Product1/1, Reshape/1  "X"
  Nomalize_noDivideByZero1/1(ehat) -> Reshape2/1  "z"
  Reshape2/1 -> Matrix Concatenate/3
  Nomalize_noDivideByZero/1(ehat) -> Cross Product1/2

== system orbit_propagator_matlab2023b/Subsystem/Attitude/changes with altitude/q (z in r) ==
  note: sc_z=-T_pos(ii,:)/norm(T_pos(ii,:));
      | sc_y=cross(sc_z,T_vel(ii,:));
      | sc_y=sc_y/norm(sc_y);
      | sc_x=cross(sc_y,sc_z);
      | sc_x=sc_x/norm(sc_x);
  posECI : Inport
  velECI : Inport  Port=2
  -1 : Gain  Gain=-1
  Cross Product : matrix_library/Cross Product
  Cross Product1 : matrix_library/Cross Product
  Direction Cosine Matrix to Quaternions : sharedtransform/Direction Cosine Matrix  to Quaternions  aMode=0  action=None  tolerance=eps(2)
      settings: LibrarySourceBlock=|
      | aerolibtransform2/Direction Cosine Matrix
      | to Quaternions
  Matrix Concatenate : Concatenate  NumInputs=3  Mode=Multidimensional array
  Nomalize_noDivideByZero : Subsystem
      mask Display: disp('u/||u||')
  Nomalize_noDivideByZero2 : Subsystem
      mask Display: disp('u/||u||')
  Nomalize_noDivideByZero4 : Subsystem
      mask Display: disp('u/||u||')
  x : Reshape  OutputDimensionality=Row vector (2-D)
  y : Reshape  OutputDimensionality=Row vector (2-D)
  z : Reshape  OutputDimensionality=Row vector (2-D)
  qECI2slor : Outport  InitialOutput=0
  amECI2slor1 : Outport  Port=2  InitialOutput=0
  wires:
  -1/1 -> Cross Product1/2, z/1, Cross Product/1  "Zslo"
  posECI/1 -> Nomalize_noDivideByZero/1(e)
  Nomalize_noDivideByZero/1(ehat) -> -1/1
  velECI/1 -> Nomalize_noDivideByZero2/1(e)
  Nomalize_noDivideByZero2/1(ehat) -> Cross Product/2
  Cross Product/1 -> Nomalize_noDivideByZero4/1(e)
  Nomalize_noDivideByZero4/1(ehat) -> Cross Product1/1, y/1  "Yslo"
  Cross Product1/1 -> x/1
  x/1 -> Matrix Concatenate/1
  y/1 -> Matrix Concatenate/2
  z/1 -> Matrix Concatenate/3
  Direction Cosine Matrix to Quaternions/1 -> qECI2slor/1
  Matrix Concatenate/1 -> amECI2slor1/1, Direction Cosine Matrix to Quaternions/1

== system orbit_propagator_matlab2023b/Subsystem/Attitude/changes with altitude/q (z in v) ==
  posECI : Inport
  velECI : Inport  Port=2
  Cross Product : matrix_library/Cross Product
  Cross Product1 : matrix_library/Cross Product
  Direction Cosine Matrix to Quaternions : sharedtransform/Direction Cosine Matrix  to Quaternions  aMode=0  action=None  tolerance=eps(2)
      settings: LibrarySourceBlock=|
      | aerolibtransform2/Direction Cosine Matrix
      | to Quaternions
  Matrix Concatenate : Concatenate  NumInputs=3  Mode=Multidimensional array
  Nomalize_noDivideByZero : Subsystem
      mask Display: disp('u/||u||')
  Nomalize_noDivideByZero2 : Subsystem
      mask Display: disp('u/||u||')
  Nomalize_noDivideByZero4 : Subsystem
      mask Display: disp('u/||u||')
  Reshape : Reshape  OutputDimensionality=Row vector (2-D)
  Reshape1 : Reshape  OutputDimensionality=Row vector (2-D)
  Reshape2 : Reshape  OutputDimensionality=Row vector (2-D)
  qECI2scbv : Outport  InitialOutput=0
  amECI2scbv : Outport  Port=2  InitialOutput=0
  wires:
  posECI/1 -> Nomalize_noDivideByZero/1(e)
  Nomalize_noDivideByZero/1(ehat) -> Cross Product/2
  velECI/1 -> Nomalize_noDivideByZero2/1(e)
  Nomalize_noDivideByZero2/1(ehat) -> Cross Product/1, Cross Product1/2, Reshape2/1  "zslo"
  Cross Product/1 -> Nomalize_noDivideByZero4/1(e)
  Nomalize_noDivideByZero4/1(ehat) -> Cross Product1/1, Reshape1/1  "Yslo"
  Reshape/1 -> Matrix Concatenate/1
  Reshape1/1 -> Matrix Concatenate/2
  Reshape2/1 -> Matrix Concatenate/3
  Direction Cosine Matrix to Quaternions/1 -> qECI2scbv/1
  Cross Product1/1 -> Reshape/1
  Matrix Concatenate/1 -> amECI2scbv/1, Direction Cosine Matrix to Quaternions/1

== system orbit_propagator_matlab2023b/Subsystem/Attitude/q (z in r)/Nomalize_noDivideByZero ==
  e : Inport
  2-norm : Subsystem
      mask Display: disp('||u||')
  Product : Product  Inputs=*/  InputSameDT=on  RndMeth=Zero  SaturateOnIntegerOverflow=on  OutDataTypeStr=Inherit: Same as first input
  Switch : Switch  Criteria=u2 > Threshold  SaturateOnIntegerOverflow=off  InputSameDT=off
  zero : Constant  Value=0
  ehat : Outport
  wires:
  e/1 -> 2-norm/1(In1), Product/1
  2-norm/1(Out1) -> Switch/2, Product/2
  Switch/1 -> ehat/1
  Product/1 -> Switch/1
  zero/1 -> Switch/3

== system orbit_propagator_matlab2023b/Subsystem/Attitude/q (z in r)/Nomalize_noDivideByZero2 ==
  e : Inport
  2-norm : Subsystem
      mask Display: disp('||u||')
  Product : Product  Inputs=*/  InputSameDT=on  RndMeth=Zero  SaturateOnIntegerOverflow=on  OutDataTypeStr=Inherit: Same as first input
  Switch : Switch  Criteria=u2 > Threshold  SaturateOnIntegerOverflow=off  InputSameDT=off
  zero : Constant  Value=0
  ehat : Outport
  wires:
  e/1 -> 2-norm/1(In1), Product/1
  2-norm/1(Out1) -> Switch/2, Product/2
  Switch/1 -> ehat/1
  Product/1 -> Switch/1
  zero/1 -> Switch/3

== system orbit_propagator_matlab2023b/Subsystem/Attitude/q (z in r)/Nomalize_noDivideByZero4 ==
  e : Inport
  2-norm : Subsystem
      mask Display: disp('||u||')
  Product : Product  Inputs=*/  InputSameDT=on  RndMeth=Zero  SaturateOnIntegerOverflow=on  OutDataTypeStr=Inherit: Same as first input
  Switch : Switch  Criteria=u2 > Threshold  SaturateOnIntegerOverflow=off  InputSameDT=off
  zero : Constant  Value=0
  ehat : Outport
  wires:
  e/1 -> 2-norm/1(In1), Product/1
  2-norm/1(Out1) -> Switch/2, Product/2
  Switch/1 -> ehat/1
  Product/1 -> Switch/1
  zero/1 -> Switch/3

== system orbit_propagator_matlab2023b/Subsystem/sun pointing in orbit plane/Nomalize_noDivideByZero1/2-norm ==
  In1 : Inport
  Math Function : Math  Operator=sqrt  SignedPower=on
  Product1 : Product  InputSameDT=on  RndMeth=Zero  SaturateOnIntegerOverflow=on  OutDataTypeStr=Inherit: Same as first input
  Sum : Sum  Inputs=+  InputSameDT=on  SaturateOnIntegerOverflow=on  OutDataTypeStr=Inherit: Same as first input
  Out1 : Outport
  wires:
  In1/1 -> Product1/1, Product1/2
  Product1/1 -> Sum/1
  Sum/1 -> Math Function/1
  Math Function/1 -> Out1/1

== system orbit_propagator_matlab2023b/Subsystem/sun pointing in orbit plane/Nomalize_noDivideByZero3/2-norm ==
  In1 : Inport
  Math Function : Math  Operator=sqrt  SignedPower=on
  Product1 : Product  InputSameDT=on  RndMeth=Zero  SaturateOnIntegerOverflow=on  OutDataTypeStr=Inherit: Same as first input
  Sum : Sum  Inputs=+  InputSameDT=on  SaturateOnIntegerOverflow=on  OutDataTypeStr=Inherit: Same as first input
  Out1 : Outport
  wires:
  In1/1 -> Product1/1, Product1/2
  Product1/1 -> Sum/1
  Sum/1 -> Math Function/1
  Math Function/1 -> Out1/1

== system orbit_propagator_matlab2023b/spare systems/create custom sun vector/Nomalize_noDivideByZero1/2-norm ==
  In1 : Inport
  Math Function : Math  Operator=sqrt  SignedPower=on
  Product1 : Product  InputSameDT=on  RndMeth=Zero  SaturateOnIntegerOverflow=on  OutDataTypeStr=Inherit: Same as first input
  Sum : Sum  Inputs=+  InputSameDT=on  SaturateOnIntegerOverflow=on  OutDataTypeStr=Inherit: Same as first input
  Out1 : Outport
  wires:
  In1/1 -> Product1/1, Product1/2
  Product1/1 -> Sum/1
  Sum/1 -> Math Function/1
  Math Function/1 -> Out1/1

== system orbit_propagator_matlab2023b/spare systems/create custom sun vector/Nomalize_noDivideByZero2/2-norm ==
  In1 : Inport
  Math Function : Math  Operator=sqrt  SignedPower=on
  Product1 : Product  InputSameDT=on  RndMeth=Zero  SaturateOnIntegerOverflow=on  OutDataTypeStr=Inherit: Same as first input
  Sum : Sum  Inputs=+  InputSameDT=on  SaturateOnIntegerOverflow=on  OutDataTypeStr=Inherit: Same as first input
  Out1 : Outport
  wires:
  In1/1 -> Product1/1, Product1/2
  Product1/1 -> Sum/1
  Sum/1 -> Math Function/1
  Math Function/1 -> Out1/1

== system orbit_propagator_matlab2023b/spare systems/sun_angle_slo/Nomalize_noDivideByZero/2-norm ==
  In1 : Inport
  Math Function : Math  Operator=sqrt  SignedPower=on
  Product1 : Product  InputSameDT=on  RndMeth=Zero  SaturateOnIntegerOverflow=on  OutDataTypeStr=Inherit: Same as first input
  Sum : Sum  Inputs=+  InputSameDT=on  SaturateOnIntegerOverflow=on  OutDataTypeStr=Inherit: Same as first input
  Out1 : Outport
  wires:
  In1/1 -> Product1/1, Product1/2
  Product1/1 -> Sum/1
  Sum/1 -> Math Function/1
  Math Function/1 -> Out1/1
